simulink model "Design2simulinka"  (R2023a)
settings: Solver=VariableStepAuto  StartTime=0.0  StopTime=1500  RelTol=1e-3
libraries: simulink x1, slpidlib x1
settings Model: Creator=anbos17  LastModifiedBy=mldro
settings RTWCC: GPUComputeCapability=5.0

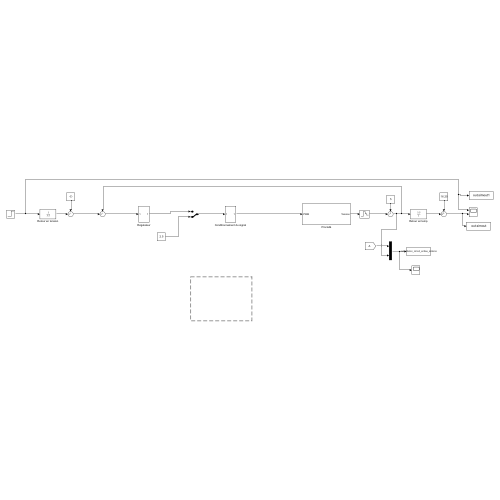
[thumbnail: Simulink's stored preview of the top-level diagram]
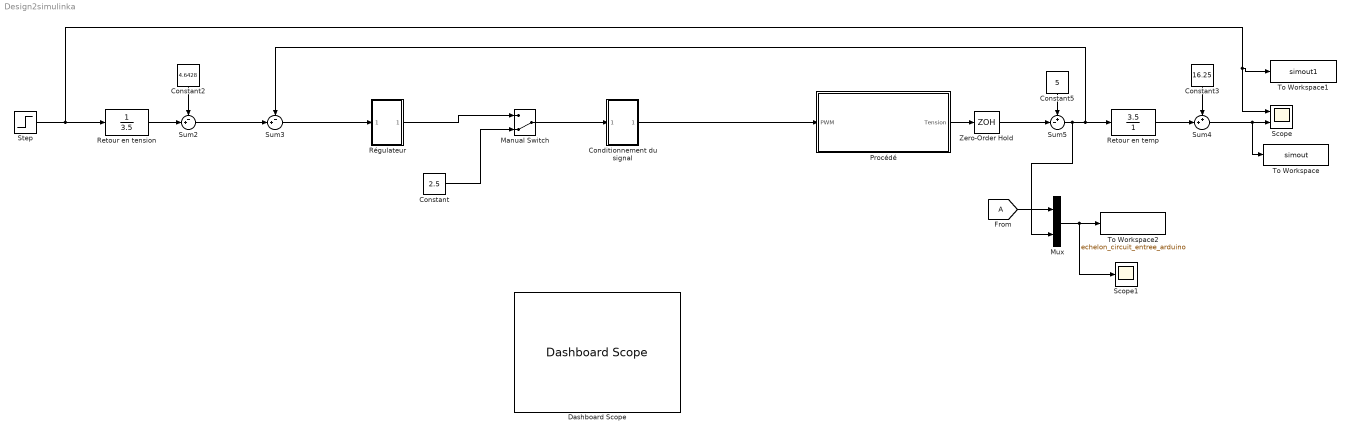
== system Design2simulinka ==
  Conditionnement du signal : Subsystem
  Constant : Constant  Value=2.5
  Constant2 : Constant  Value=4.6428
  Constant3 : Constant  Value=16.25
  Constant5 : Constant  Value=5
  Dashboard Scope : DashboardScope
  From : From  TagVisibility=global
  Manual Switch : ManualSwitch  CurrentSetting=0
  Mux : Mux  Inputs=2
  Procédé : Subsystem
  Retour en temp : TransferFcn  Numerator=[3.5]  Denominator=[1]
  Retour en tension : TransferFcn  Denominator=[3.5]
  Régulateur : Subsystem
  Scope : Scope  NumInputPorts=2
  Scope1 : Scope
  Step : Step  Time=600  Before=25  After=28  SampleTime=0
  Sum2 : Sum  Inputs=-+|  InputSameDT=on  SaturateOnIntegerOverflow=on  OutDataTypeStr=Inherit: Same as first input
  Sum3 : Sum  Inputs=-+|  InputSameDT=on  SaturateOnIntegerOverflow=on  OutDataTypeStr=Inherit: Same as first input
  Sum4 : Sum  Inputs=++|  InputSameDT=on  SaturateOnIntegerOverflow=on  OutDataTypeStr=Inherit: Same as first input
  Sum5 : Sum  Inputs=+-|  InputSameDT=on  SaturateOnIntegerOverflow=on  OutDataTypeStr=Inherit: Same as first input
  To Workspace : ToWorkspace  VariableName=simout  SaveFormat=Structure With Time  SampleTime=-1
  To Workspace1 : ToWorkspace  VariableName=simout1  SampleTime=-1
  To Workspace2 : ToWorkspace  VariableName=echelon_circuit_entree_arduino  SampleTime=1
  Zero-Order Hold : ZeroOrderHold
  wires:
  Retour en temp/1 -> Sum4/2
  Constant3/1 -> Sum4/1
  Constant5/1 -> Sum5/1
  Sum5/1 -> Mux/2, Sum3/1, Retour en temp/1
  Step/1 -> Retour en tension/1, To Workspace1/1, Scope/1
  Constant2/1 -> Sum2/1
  Retour en tension/1 -> Sum2/2
  Procédé/1(Tension) -> Zero-Order Hold/1
  Zero-Order Hold/1 -> Sum5/2
  Sum4/1 -> To Workspace/1, Scope/2
  Sum2/1 -> Sum3/2
  Sum3/1 -> Régulateur/1(In1)
  Conditionnement du signal/1(Out1) -> Procédé/1(PWM)
  From/1 -> Mux/1
  Mux/1 -> To Workspace2/1, Scope1/1
  Manual Switch/1 -> Conditionnement du signal/1(In1)
  Régulateur/1(Out1) -> Manual Switch/1
  Constant/1 -> Manual Switch/2

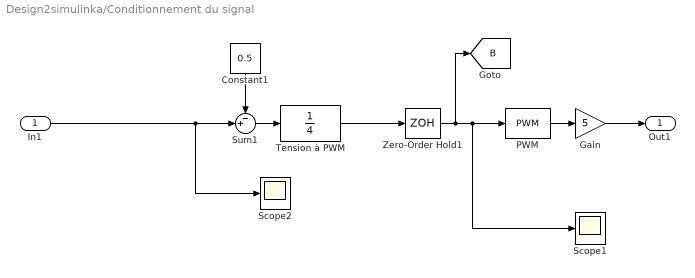
== system Design2simulinka/Conditionnement du signal ==
  In1 : Inport
  Constant1 : Constant  Value=0.5
  Gain : Gain  Gain=5
  PWM : simulink/Discontinuities/PWM  DisableCoverage=on  Period=0.002048  InitialDelay=0  DisallowZeroDutyCycle=off  RunAtFixedTimeIntervals=off  SampleTime=0.1
  Scope1 : Scope
  Scope2 : Scope
  Sum1 : Sum  Inputs=-+|  InputSameDT=on  SaturateOnIntegerOverflow=on  OutDataTypeStr=Inherit: Same as first input
  Tension à PWM : TransferFcn  Denominator=[4]
  Zero-Order Hold1 : ZeroOrderHold
  Out1 : Outport
  tag scope: B=global
  wires:
  PWM/1 -> Gain/1
  Zero-Order Hold1/1 -> [B], PWM/1, Scope1/1
  In1/1 -> Scope2/1, Sum1/2
  Constant1/1 -> Sum1/1
  Gain/1 -> Out1/1
  Sum1/1 -> Tension à PWM/1
  Tension à PWM/1 -> Zero-Order Hold1/1

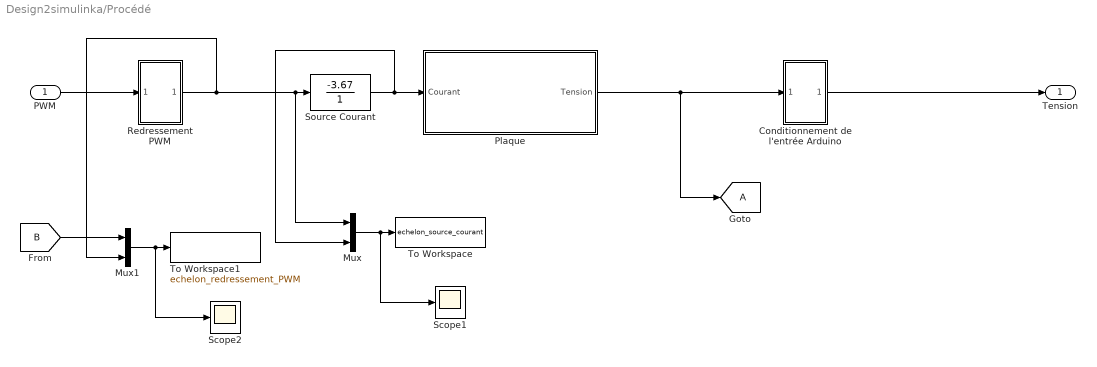
== system Design2simulinka/Procédé ==
  PWM : Inport
  Conditionnement de l'entrée Arduino : Subsystem
  Goto : Goto  TagVisibility=global
  Mux : Mux  Inputs=2
  Mux1 : Mux  Inputs=2
  Plaque : Subsystem
  Redressement PWM : Subsystem
  Scope1 : Scope
  Scope2 : Scope
  Source Courant : TransferFcn  Numerator=[-3.67]  Denominator=[1]
  To Workspace : ToWorkspace  VariableName=echelon_source_courant  SampleTime=1
  To Workspace1 : ToWorkspace  VariableName=echelon_redressement_PWM  SampleTime=1
  Tension : Outport
  wires:
  Source Courant/1 -> Mux/2, Plaque/1(Courant)
  PWM/1 -> Redressement PWM/1(In1)
  Redressement PWM/1(Out1) -> Mux1/2, Mux/1, Source Courant/1
  Plaque/1(Tension) -> Conditionnement de l'entrée Arduino/1(In1), Goto/1
  Conditionnement de l'entrée Arduino/1(Out1) -> Tension/1
  Mux/1 -> Scope1/1, To Workspace/1
  Mux1/1 -> Scope2/1, To Workspace1/1
  [B] -> Mux1/1

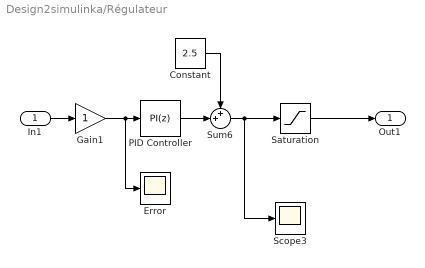
== system Design2simulinka/Régulateur ==
  In1 : Inport
  Constant : Constant  Value=2.5
  Error : Scope
  Gain1 : Gain
  PID Controller : slpidlib/PID Controller  Controller=PI  Form=Parallel  TimeDomain=Discrete-time  UseExternalTs=off  SampleTime=1  IntegratorMethod=Forward Euler  FilterMethod=Forward Euler  ControllerParametersSource=internal  P=0.53  I=0.0049  UseKiTs=off  D=20.0097  N=4.5847  UseFilter=on  TunerSelectOption=Transfer Function Based (PID Tuner App)  InitialConditionSource=internal  InitialConditionForIntegrator=0  InitialConditionForFilter=0  DifferentiatorICPrevScaledInput=0  ExternalReset=none  TrackingMode=off  Kt=1  LimitOutput=off  SatLimitsSource=internal  UpperSaturationLimit=inf  LowerSaturationLimit=-inf  LinearizeAsGain=on  AntiWindupMode=none  Kb=1  LimitIntegrator=off  UpperIntegratorSaturationLimit=inf  LowerIntegratorSaturationLimit=-inf  POutMin=[]  POutMax=[]  IOutMin=[]  IOutMax=[]  DOutMin=[]  DOutMax=[]  NOutMin=[]  NOutMax=[]  SumOutMin=[]  SumOutMax=[]  SaturationOutMin=[]  SaturationOutMax=[]  PParamMin=[]  PParamMax=[]  IParamMin=[]  IParamMax=[]  DParamMin=[]  DParamMax=[]  NParamMin=[]  NParamMax=[]  KbParamMin=[]  KbParamMax=[]  KtParamMin=[]  KtParamMax=[]  KbOutMin=[]  KbOutMax=[]  KtOutMin=[]  KtOutMax=[]  IntegratorOutMin=[]  IntegratorOutMax=[]  FilterOutMin=[]  FilterOutMax=[]  SumI1OutMin=[]  SumI1OutMax=[]  SumI2OutMin=[]  SumI2OutMax=[]  SumI3OutMin=[]  SumI3OutMax=[]  SumI4OutMin=[]  SumI4OutMax=[]  SumDOutMin=[]  SumDOutMax=[]  DifferentiatorOutMin=[]  DifferentiatorOutMax=[]  FilterDiffOutCoefMin=[]  FilterDiffOutCoefMax=[]  ReciprocalOutMin=[]  ReciprocalOutMax=[]  SumDenOutMin=[]  SumDenOutMax=[]  SumNumOutMin=[]  SumNumOutMax=[]  DivideOutMin=[]  DivideOutMax=[]  UdiffTsProdOutMin=[]  UdiffTsProdOutMax=[]  NTsProdOutMin=[]  NTsProdOutMax=[]  UintegralTsProdOutMin=[]  UintegralTsProdOutMax=[]  UngainTsProdOutMin=[]  UngainTsProdOutMax=[]  ClampingZeroOutDataTypeStr=Inherit: Inherit via back propagation  ClampingZeroOutMin=[]  ClampingZeroOutMax=[]  FilterDenConstantOutDataTypeStr=Inherit: Inherit via back propagation  FilterDenConstantOutMin=[]  FilterDenConstantOutMax=[]  PCopyOutDataTypeStr=Inherit: Inherit via back propagation  PCopyOutMin=[]  PCopyOutMax=[]  NCopyOutDataTypeStr=Inherit: Inherit via back propagation  NCopyOutMin=[]  NCopyOutMax=[]  IntegratorContinuousStateAttributes=''  IntegratorStateMustResolveToSignalObject=off  IntegratorRTWStateStorageClass=Auto  FilterContinuousStateAttributes=''  FilterStateMustResolveToSignalObject=off  FilterRTWStateStorageClass=Auto  ParallelPVariant=InternalParameters  IdealPVariant=Disabled  IVariant=InternalParameters  DVariant=Disabled  IntegratorVariant=Discrete  SatVariant=Disabled  AWVariant=Passthrough  PCopyVariant=Disabled  TRVariant=Disabled  FdbkBlocksVariant=Forward  IdealPFdbkVariant=Disabled  SatFdbkVariant=Disabled  DerivativeFilterVariant=Disabled  NVariant=Disabled  NCopyVariant=Disabled_SignalSpec  FilterICVariant=Disabled  IntegratorICVariant=InternalICs  ExternalResetVariant=Disabled  TRSumVariant=Passthrough  SumFdbkVariant=Disabled  SumVariant=Sum_PI  TsampFilterVariant=InternalTs  TsampNgainVariant=Passthrough  TsampIntegralVariant=Disabled_SignalSpec  ExternalSaturationOutDataTypeStr=Inherit: Same as second input
  Saturation : Saturate  UpperLimit=4.9  LowerLimit=0.1
  Scope3 : Scope
  Sum6 : Sum  Inputs=++|  InputSameDT=on  SaturateOnIntegerOverflow=on  OutDataTypeStr=Inherit: Same as first input
  Out1 : Outport
  wires:
  Constant/1 -> Sum6/1
  PID Controller/1 -> Sum6/2
  Gain1/1 -> Error/1, PID Controller/1
  Sum6/1 -> Saturation/1, Scope3/1
  Saturation/1 -> Out1/1
  In1/1 -> Gain1/1

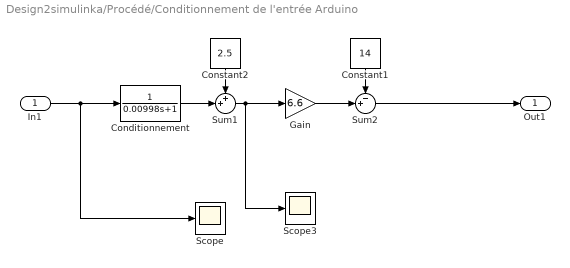
== system Design2simulinka/Procédé/Conditionnement de l'entrée Arduino ==
  In1 : Inport
  Conditionnement : TransferFcn  Denominator=[0.00998 1]
  Constant1 : Constant  Value=14
  Constant2 : Constant  Value=2.5
  Gain : Gain  Gain=6.6
  Scope : Scope
  Scope3 : Scope
  Sum1 : Sum  Inputs=++|  InputSameDT=on  SaturateOnIntegerOverflow=on  OutDataTypeStr=Inherit: Same as first input
  Sum2 : Sum  Inputs=-+|  InputSameDT=on  SaturateOnIntegerOverflow=on  OutDataTypeStr=Inherit: Same as first input
  Out1 : Outport
  wires:
  Constant1/1 -> Sum2/1
  Gain/1 -> Sum2/2
  Constant2/1 -> Sum1/1
  Sum2/1 -> Out1/1
  Conditionnement/1 -> Sum1/2
  Sum1/1 -> Gain/1, Scope3/1
  In1/1 -> Conditionnement/1, Scope/1

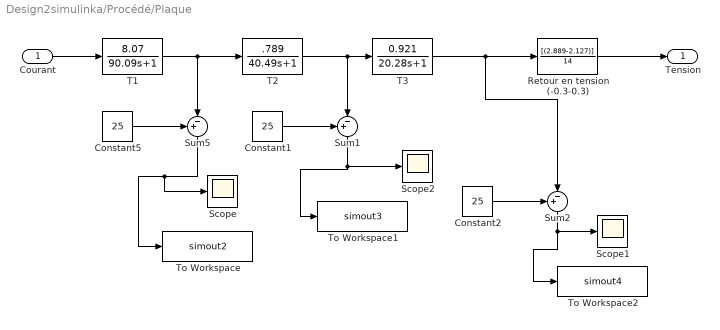
== system Design2simulinka/Procédé/Plaque ==
  Courant : Inport
  Constant1 : Constant  Value=25
  Constant2 : Constant  Value=25
  Constant5 : Constant  Value=25
  Retour en tension (-0.3-0.3) : TransferFcn  Numerator=[(2.889-2.127)]  Denominator=[14]
  Scope : Scope
  Scope1 : Scope
  Scope2 : Scope
  Sum1 : Sum  Inputs=+-|  InputSameDT=on  SaturateOnIntegerOverflow=on  OutDataTypeStr=Inherit: Same as first input
  Sum2 : Sum  Inputs=+-|  InputSameDT=on  SaturateOnIntegerOverflow=on  OutDataTypeStr=Inherit: Same as first input
  Sum5 : Sum  Inputs=+-|  InputSameDT=on  SaturateOnIntegerOverflow=on  OutDataTypeStr=Inherit: Same as first input
  T1 : TransferFcn  Numerator=8.07  Denominator=[90.09 1]
  T2 : TransferFcn  Numerator=.789  Denominator=[40.49 1]
  T3 : TransferFcn  Numerator=0.921  Denominator=[20.28 1]
  To Workspace : ToWorkspace  VariableName=simout2  SaveFormat=Timeseries  SampleTime=-1
  To Workspace1 : ToWorkspace  VariableName=simout3  SaveFormat=Timeseries  SampleTime=-1
  To Workspace2 : ToWorkspace  VariableName=simout4  SaveFormat=Timeseries  SampleTime=-1
  Tension : Outport
  wires:
  Courant/1 -> T1/1
  T1/1 -> Sum5/2, T2/1
  T2/1 -> T3/1, Sum1/2
  T3/1 -> Retour en tension (-0.3-0.3)/1, Sum2/2
  Retour en tension (-0.3-0.3)/1 -> Tension/1
  Constant5/1 -> Sum5/1
  Sum5/1 -> To Workspace/1, Scope/1
  Sum1/1 -> To Workspace1/1, Scope2/1
  Constant1/1 -> Sum1/1
  Sum2/1 -> To Workspace2/1, Scope1/1
  Constant2/1 -> Sum2/1

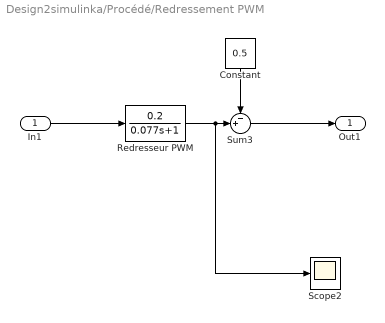
== system Design2simulinka/Procédé/Redressement PWM ==
  In1 : Inport
  Constant : Constant  Value=0.5
  Redresseur PWM : TransferFcn  Numerator=[0.2]  Denominator=[0.077 1]
  Scope2 : Scope
  Sum3 : Sum  Inputs=-+|  InputSameDT=on  SaturateOnIntegerOverflow=on  OutDataTypeStr=Inherit: Same as first input
  Out1 : Outport
  wires:
  Redresseur PWM/1 -> Scope2/1, Sum3/2
  Sum3/1 -> Out1/1
  Constant/1 -> Sum3/1
  In1/1 -> Redresseur PWM/1
